simulink model "simul_off_on_control"  (R2019a)
settings: Solver=ode4  StartTime=0.0  StopTime=500  FixedStep=0.1  RelTol=1e-3  EnableMultiTasking=on
StartFcn:
  | clear all
values from neighbouring files (symbols this model uses):
  K = M1.Kp    [ident_via_contsid.m]
  T = M1.Tp1    [ident_via_contsid.m]    (also in test_your_model.m)
  tau = M1.Td    [ident_via_contsid.m]    (also in test_your_model.m)
settings Model: Creator=johnh  LastModifiedBy=hgarnier
settings DataIOCC: ReturnWorkspaceOutputs=off
settings OptimizationCC: LifeSpan=inf
settings DebuggingCC: PregeneratedLibrarySubsystemCodeDiagnostic=none  SFUnexpectedBacktrackingDiag=warning  SFNoUnconditionalDefaultTransitionDiag=warning  SFExecutionAtInitializationDiag=none  ArithmeticOperatorsInVariantConditions=warning
settings SFSimCC: SimUseLocalCustomCode=off
settings RTWCC: RTWUseLocalCustomCode=off
settings CodeAppCC: StateflowObjectComments=on
settings GRTTargetCC: TargetLangStandard=C89/C90 (ANSI)  GeneratePreprocessorConditionals=Disable all
settings ConfigComp: CovMetricSettings=dw  CovHtmlReporting=on  CovSaveCumulativeToWorkspaceVar=on  CovSaveSingleToWorkspaceVar=on  CovExternalEMLEnable=off

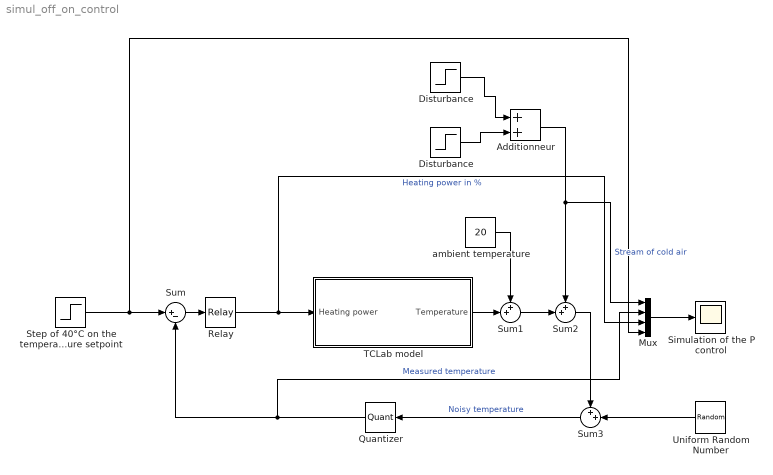
== system simul_off_on_control ==
  Additionneur : Sum
  Disturbance : Step  Time=300  After=-3  SampleTime=0
  "Disturbance " : Step  Time=320  After=+3  SampleTime=0
  Mux : Mux
  Quantizer : Quantizer  QuantizationInterval=0.4
  Relay : Relay  OffSwitchValue=-eps  OnOutputValue=100
  Simulation of the P control : Scope
  Step of 40°C on the temperature setpoint : Step  Time=20  After=40  SampleTime=0
  Sum : Sum  Inputs=|+-
  Sum1 : Sum  Inputs=++|
  Sum2 : Sum  Inputs=++|
  Sum3 : Sum  Inputs=++|
  TCLab model : Subsystem
  Uniform Random Number : UniformRandomNumber  Minimum=-0.8  Maximum=0.4  SampleTime=0.1
  "ambient temperature " : Constant  Value=20
  wires:
  Mux/1 -> Simulation of the P control/1
  Step of 40°C on the temperature setpoint/1 -> Mux/4, Sum/1
  Sum/1 -> Relay/1
  "ambient temperature "/1 -> Sum1/1
  Relay/1 -> Mux/3, TCLab model/1("Heating power ")  "Heating power in %"
  TCLab model/1("Temperature ") -> Sum1/2
  Sum1/1 -> Sum2/2
  Sum2/1 -> Sum3/1
  Disturbance/1 -> Additionneur/1
  "Disturbance "/1 -> Additionneur/2
  Additionneur/1 -> Mux/1, Sum2/1  "Stream of cold air"
  Sum3/1 -> Quantizer/1  "Noisy temperature"
  Uniform Random Number/1 -> Sum3/2
  Quantizer/1 -> Mux/2, Sum/2  "Measured temperature"

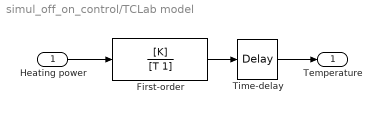
== system simul_off_on_control/TCLab model ==
  "Heating power " : Inport
  First-order : TransferFcn  Numerator=[K]  Denominator=[T 1]
  Time-delay : TransportDelay  DelayTime=tau
  "Temperature " : Outport
  wires:
  "Heating power "/1 -> First-order/1
  First-order/1 -> Time-delay/1
  Time-delay/1 -> "Temperature "/1
